simulink model "lunland"  (Simulink 2.20)
settings: Solver=ode45  StartTime=0.0  StopTime=400  MaxStep=0.5  RelTol=1e-3  AbsTol=1e-3
values from neighbouring files (symbols this model uses):
  c1 = 2.77e-4    (= 0.000277)    [LVSTMOND.M]
  c2 = 4.925e12    (= 4925000000000)    [LVSTMOND.M]
  F1 = 36350    [LVSTMOND.M]
  F2 = 1308    [LVSTMOND.M]
  h0 = 59404    [LVSTMOND.M]
  m0 = 1038.358    [LVSTMOND.M]
  r = 1738000    [LVSTMOND.M]
  T1 = 43.2    [LVSTMOND.M]
  T2 = 210    [LVSTMOND.M]
  v0 = -2003    [LVSTMOND.M]
libraries: simulink x1
settings Model: SaveTime=off  SaveOutput=off  ConsistencyChecking=off  RTWPlaceOutputsASAP=off

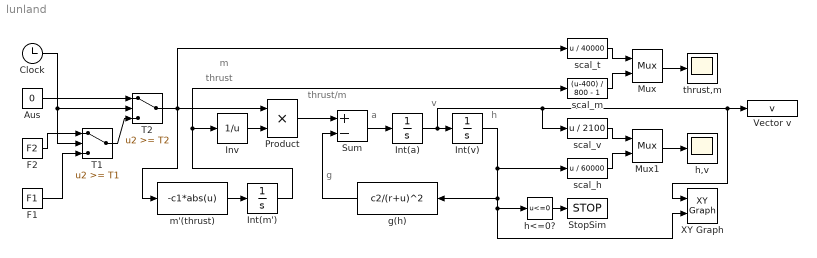
== system lunland ==
  note: a
  note: thrust/m
  note: g
  note: h
  note: v
  note: thrust
  note: m
  Aus : Constant  Value=0
  Clock : Clock
  F1 : Constant  Value=F1
  F2 : Constant  Value=F2
  Int(a) : Integrator  ExternalReset=none  InitialConditionSource=internal  InitialCondition=v0  LimitOutput=off  UpperSaturationLimit=inf  LowerSaturationLimit=-inf  ShowSaturationPort=off  ShowStatePort=off  AbsoluteTolerance=auto
  Int(m') : Integrator  ExternalReset=none  InitialConditionSource=internal  InitialCondition=m0  LimitOutput=off  UpperSaturationLimit=inf  LowerSaturationLimit=-inf  ShowSaturationPort=off  ShowStatePort=off  AbsoluteTolerance=auto
  Int(v) : Integrator  ExternalReset=none  InitialConditionSource=internal  InitialCondition=h0  LimitOutput=off  UpperSaturationLimit=inf  LowerSaturationLimit=-inf  ShowSaturationPort=off  ShowStatePort=off  AbsoluteTolerance=auto
  Inv : Fcn  Expr=1/u
  Mux : Mux  Inputs=2
  Mux1 : Mux  Inputs=2
  Product : Product  Inputs=2
  StopSim : Stop
  Sum : Sum  Inputs=+-
  T1 : Switch  Threshold=T1
  T2 : Switch  Threshold=T2
  Vector v : ToWorkspace  VariableName=v  SampleTime=0
      settings: Buffer=5000
  XY Graph : simulink/Sinks/XY Graph  xmin=-2000  xmax=0  ymin=0  ymax=60000  st=-1
  g(h) : Fcn  Orientation=left  Expr=c2/(r+u)^2
  h,v : Scope
      settings: TickLabels=on  TimeRange=250  YMin=-1  YMax=1  SaveToWorkspace=off  SaveName=ScopeData  LimitMaxRows=off
  h<=0? : Fcn  Expr=u<=0
  m'(thrust) : Fcn  Expr=-c1*abs(u)
  scal_h : Fcn  Expr=u / 60000
  scal_m : Fcn  Expr=(u-400) / 800 - 1
  scal_t : Fcn  Expr=u / 40000
  scal_v : Fcn  Expr=u / 2100
  thrust,m : Scope
      settings: TickLabels=on  TimeRange=250  YMin=-1  YMax=1  SaveToWorkspace=off  SaveName=ScopeData  LimitMaxRows=off
  wires:
  Product/1 -> Sum/1
  Inv/1 -> Product/2
  Sum/1 -> Int(a)/1
  g(h)/1 -> Sum/2
  T1/1 -> T2/3
  F1/1 -> T1/3
  F2/1 -> T1/1
  Aus/1 -> T2/1
  Clock/1 -> T1/2, T2/2
  m'(thrust)/1 -> Int(m')/1
  T2/1 -> Product/1, m'(thrust)/1, scal_t/1
  Mux/1 -> thrust,m/1
  scal_t/1 -> Mux/1
  scal_m/1 -> Mux/2
  Int(m')/1 -> Inv/1, scal_m/1
  Int(a)/1 -> Int(v)/1, scal_v/1, XY Graph/1, Vector v/1
  scal_v/1 -> Mux1/1
  scal_h/1 -> Mux1/2
  Mux1/1 -> h,v/1
  h<=0?/1 -> StopSim/1
  Int(v)/1 -> scal_h/1, h<=0?/1, XY Graph/2, g(h)/1
